simulink model "MainController"  (R2020a)
settings: Solver=VariableStepAuto  StartTime=0.0  StopTime=10.0  RelTol=1e-3
undefined symbols (not defined in the file): Angle, Ankle, Hip, Knee, Left, Right, Speed, Torque
settings Model: DataDictionary=MainControllerParameters.sldd  EnableAccessToBaseWorkspace=off  Creator=khoi  LastModifiedBy=khoi

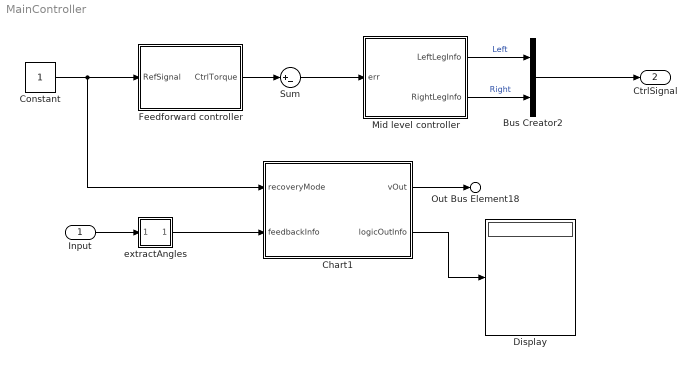
== system MainController ==
  Input : Inport  OutDataTypeStr=Bus: ExoskeletonSignal
  Bus Creator2 : BusCreator  Inputs=Left,Right  OutDataTypeStr=Bus: ExoskeletonSignal  NonVirtualBus=on
  Chart1 : Stateflow chart  TreatAsAtomicUnit=on
  Constant : Constant
  Display : Display
  Feedforward controller : Subsystem
  Mid level controller : Subsystem
  Sum : Sum  Inputs=|+-
  extractAngles : Subsystem
  Out Bus Element18 : Outport  PortName=Params  Element=vSupply
  CtrlSignal : Outport  Port=2
  wires:
  Sum/1 -> Mid level controller/1(err)
  Feedforward controller/1(CtrlTorque) -> Sum/1
  Constant/1 -> Chart1/1(recoveryMode), Feedforward controller/1(RefSignal)
  Chart1/1(vOut) -> Out Bus Element18/1
  Bus Creator2/1 -> CtrlSignal/1
  Mid level controller/2(RightLegInfo) -> Bus Creator2/2  "Right"
  Mid level controller/1(LeftLegInfo) -> Bus Creator2/1  "Left"
  Chart1/2(logicOutInfo) -> Display/1
  Input/1 -> extractAngles/1(In1)
  extractAngles/1(Out1) -> Chart1/2(feedbackInfo)

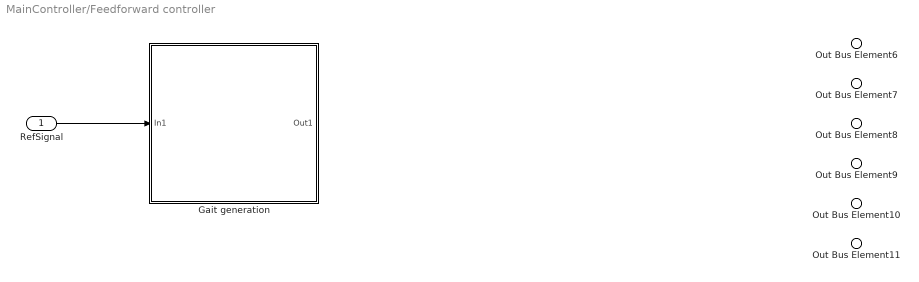
== system MainController/Feedforward controller ==
  RefSignal : Inport
  Gait generation : Subsystem
  Out Bus Element6 : Outport  PortName=CtrlTorque  Element=Left.Hip
  Out Bus Element8 : Outport  PortName=CtrlTorque  Element=Left.Knee
  Out Bus Element7 : Outport  PortName=CtrlTorque  Element=Left.Ankle
  Out Bus Element9 : Outport  PortName=CtrlTorque  Element=Right.Hip
  Out Bus Element10 : Outport  PortName=CtrlTorque  Element=Right.Knee
  Out Bus Element11 : Outport  PortName=CtrlTorque  Element=Right.Ankle
  wires:
  RefSignal/1 -> Gait generation/1(In1)

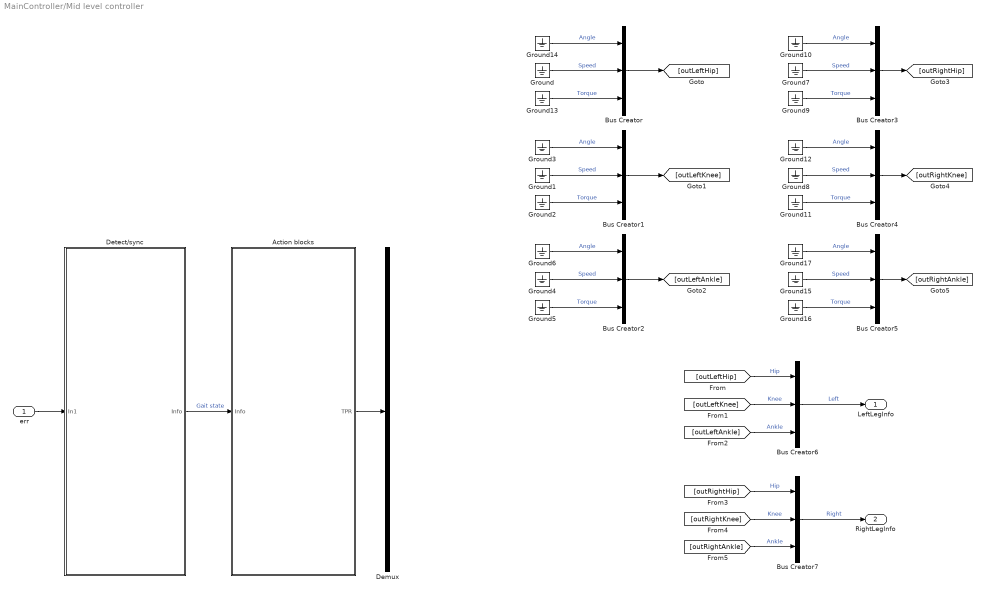
== system MainController/Mid level controller ==
  err : Inport
  Action blocks : Subsystem
  Bus Creator{,1..5} (6 alike) : BusCreator  Inputs=Angle,Speed,Torque  OutDataTypeStr=Bus: RespSignal  NonVirtualBus=on
  Bus Creator6 : BusCreator  Inputs=Hip,Knee,Ankle  OutDataTypeStr=Bus: LegSignal  NonVirtualBus=on
  Bus Creator7 : BusCreator  Inputs=Hip,Knee,Ankle  OutDataTypeStr=Bus: LegSignal  NonVirtualBus=on
  Demux : Demux  Outputs=6
  Detect/sync : Subsystem
  Ground{,1..17} (18 alike) : Ground
  LeftLegInfo : Outport
  RightLegInfo : Outport  Port=2
  wires:
  err/1 -> Detect/sync/1(In1)
  Detect/sync/1(Info) -> Action blocks/1(Info)  "Gait state"
  Action blocks/1(TPR) -> Demux/1
  Ground14/1 -> Bus Creator/1  "Angle"
  Ground/1 -> Bus Creator/2  "Speed"
  Ground13/1 -> Bus Creator/3  "Torque"
  Ground2/1 -> Bus Creator1/3  "Torque"
  Ground1/1 -> Bus Creator1/2  "Speed"
  Ground3/1 -> Bus Creator1/1  "Angle"
  Ground6/1 -> Bus Creator2/1  "Angle"
  Ground4/1 -> Bus Creator2/2  "Speed"
  Ground5/1 -> Bus Creator2/3  "Torque"
  Ground16/1 -> Bus Creator5/3  "Torque"
  Ground15/1 -> Bus Creator5/2  "Speed"
  Ground17/1 -> Bus Creator5/1  "Angle"
  Ground12/1 -> Bus Creator4/1  "Angle"
  Ground8/1 -> Bus Creator4/2  "Speed"
  Ground11/1 -> Bus Creator4/3  "Torque"
  Ground9/1 -> Bus Creator3/3  "Torque"
  Ground7/1 -> Bus Creator3/2  "Speed"
  Ground10/1 -> Bus Creator3/1  "Angle"
  Bus Creator/1 -> [outLeftHip]
  Bus Creator1/1 -> [outLeftKnee]
  Bus Creator2/1 -> [outLeftAnkle]
  Bus Creator3/1 -> [outRightHip]
  Bus Creator4/1 -> [outRightKnee]
  Bus Creator5/1 -> [outRightAnkle]
  [outLeftAnkle] -> Bus Creator6/3  "Ankle"
  [outRightHip] -> Bus Creator7/1  "Hip"
  [outLeftKnee] -> Bus Creator6/2  "Knee"
  [outLeftHip] -> Bus Creator6/1  "Hip"
  [outRightKnee] -> Bus Creator7/2  "Knee"
  [outRightAnkle] -> Bus Creator7/3  "Ankle"
  Bus Creator6/1 -> LeftLegInfo/1  "Left"
  Bus Creator7/1 -> RightLegInfo/1  "Right"

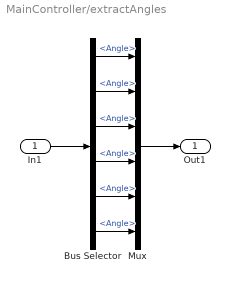
== system MainController/extractAngles ==
  In1 : Inport
  Bus Selector : BusSelector  OutputSignals=Left.Hip.Angle,Left.Knee.Angle,Left.Ankle.Angle,Right.Hip.Angle,Right.Knee.Angle,Right.Ankle.Angle
  Mux : Mux  Inputs=6
  Out1 : Outport
  wires:
  Bus Selector/4 -> Mux/4  "<Angle>"
  Bus Selector/6 -> Mux/6  "<Angle>"
  In1/1 -> Bus Selector/1
  Mux/1 -> Out1/1
  Bus Selector/1 -> Mux/1  "<Angle>"
  Bus Selector/5 -> Mux/5  "<Angle>"
  Bus Selector/3 -> Mux/3  "<Angle>"
  Bus Selector/2 -> Mux/2  "<Angle>"

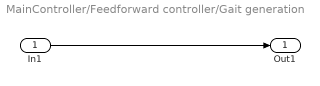
== system MainController/Feedforward controller/Gait generation ==
  In1 : Inport
  Out1 : Outport
  wires:
  In1/1 -> Out1/1

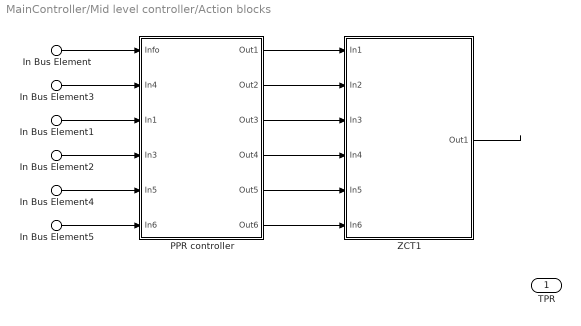
== system MainController/Mid level controller/Action blocks ==
  In Bus Element : Inport  PortName=Info  Element=Right.Hip
  In Bus Element1 : Inport  PortName=Info  Element=Right.Knee
  In Bus Element2 : Inport  PortName=Info  Element=Right.Ankle
  In Bus Element3 : Inport  PortName=Info  Element=Left.Hip
  In Bus Element4 : Inport  PortName=Info  Element=Left.Knee
  In Bus Element5 : Inport  PortName=Info  Element=Left.Ankle
  PPR controller : Subsystem
  ZCT1 : Subsystem
  TPR : Outport
  wires:
  ? -> TPR/1
  PPR controller/1(Out1) -> ZCT1/1(In1)
  ZCT1/1(Out1) -> ?
  In Bus Element/1 -> PPR controller/1(Info)
  In Bus Element3/1 -> PPR controller/2(In4)
  In Bus Element1/1 -> PPR controller/3(In1)
  In Bus Element2/1 -> PPR controller/4(In3)
  PPR controller/2(Out2) -> ZCT1/2(In2)
  PPR controller/3(Out3) -> ZCT1/3(In3)
  PPR controller/4(Out4) -> ZCT1/4(In4)
  In Bus Element4/1 -> PPR controller/5(In5)
  In Bus Element5/1 -> PPR controller/6(In6)
  PPR controller/5(Out5) -> ZCT1/5(In5)
  PPR controller/6(Out6) -> ZCT1/6(In6)

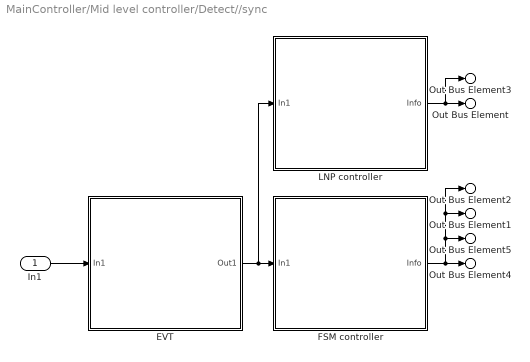
== system MainController/Mid level controller/Detect//sync ==
  In1 : Inport
  EVT : Subsystem
  FSM controller : Subsystem
  LNP controller : Subsystem
  Out Bus Element3 : Outport  PortName=Info  Element=Left.Hip
  Out Bus Element4 : Outport  PortName=Info  Element=Left.Knee
  Out Bus Element5 : Outport  PortName=Info  Element=Left.Ankle
  Out Bus Element : Outport  PortName=Info  Element=Right.Hip
  Out Bus Element1 : Outport  PortName=Info  Element=Right.Knee
  Out Bus Element2 : Outport  PortName=Info  Element=Right.Ankle
  wires:
  In1/1 -> EVT/1(In1)
  FSM controller/1(Info) -> Out Bus Element1/1, Out Bus Element2/1, Out Bus Element5/1, Out Bus Element4/1
  EVT/1(Out1) -> LNP controller/1(In1), FSM controller/1(In1)
  LNP controller/1(Info) -> Out Bus Element/1, Out Bus Element3/1

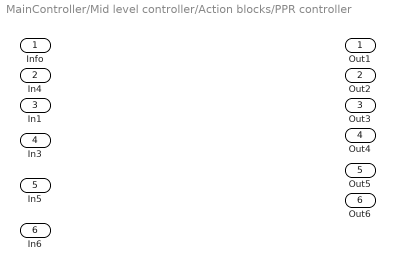
== system MainController/Mid level controller/Action blocks/PPR controller ==
  Info : Inport
  In4 : Inport  Port=2
  In1 : Inport  Port=3
  In3 : Inport  Port=4
  In5 : Inport  Port=5
  In6 : Inport  Port=6
  Out1 : Outport
  Out2 : Outport  Port=2
  Out3 : Outport  Port=3
  Out4 : Outport  Port=4
  Out5 : Outport  Port=5
  Out6 : Outport  Port=6

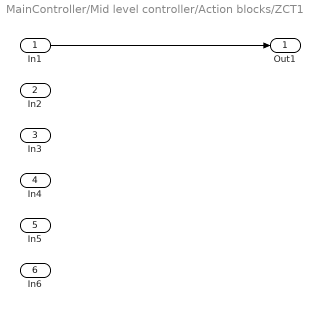
== system MainController/Mid level controller/Action blocks/ZCT1 ==
  In1 : Inport
  In2 : Inport  Port=2
  In3 : Inport  Port=3
  In4 : Inport  Port=4
  In5 : Inport  Port=5
  In6 : Inport  Port=6
  Out1 : Outport
  wires:
  In1/1 -> Out1/1

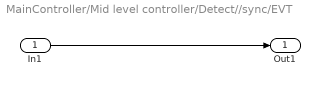
== system MainController/Mid level controller/Detect//sync/EVT ==
  In1 : Inport
  Out1 : Outport
  wires:
  In1/1 -> Out1/1

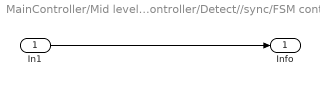
== system MainController/Mid level controller/Detect//sync/FSM controller ==
  In1 : Inport
  Info : Outport
  wires:
  In1/1 -> Info/1

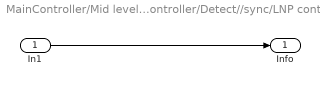
== system MainController/Mid level controller/Detect//sync/LNP controller ==
  In1 : Inport
  Info : Outport
  wires:
  In1/1 -> Info/1

== stateflow chart MainController/Chart1 ==
  state SITTING [group] [commented out]
  state GoToSitting [commented out]
  state ReadyForStandingUp [commented out]
  state InitParams
    entry:
    state voltageSupplyModifier
      (default) -> (junction 332) : % Control on patient's mobility
      (junction 332) -> (junction 333) [order 1] : [recoveryMode == 1]
      (junction 332) -> (junction 321) [order 2]
      (junction 333) -> (junction 334) : {vOut = 0.2*Vsup;}
      (junction 334) -> (junction 331)
      (junction 331) -> (junction 323)
      (junction 321) -> (junction 322) [order 1] : [recoveryMode == 2]
      (junction 321) -> (junction 325) [order 2]
      (junction 322) -> (junction 335) : {vOut = 0.4*Vsup;}
      (junction 335) -> (junction 323)
      (junction 323) -> (junction 319)
      (junction 325) -> (junction 326) [order 1] : [recoveryMode == 3]
      (junction 325) -> (junction 320) [order 2]
      (junction 326) -> (junction 328) : {vOut = 0.6*Vsup;}
      (junction 328) -> (junction 319)
      (junction 319) -> (junction 351)
      (junction 320) -> (junction 329) [order 1] : [recoveryMode == 4]
      (junction 320) -> (junction 350) [order 2]
      (junction 329) -> (junction 330) : {vOut = 0.8*Vsup;}
      (junction 330) -> (junction 351)
      (junction 351) -> (junction 349)
      (junction 350) -> (junction 352) [order 1] : [recoveryMode == 5]
      (junction 350) -> (junction 353) [order 2] : {vOut = 0;}
      (junction 352) -> (junction 346) : {vOut = 1.0*Vsup;}
      (junction 346) -> (junction 349)
      (junction 349) -> (junction 354)
      (junction 354) -> (junction 353)
      (junction 353) -> (junction 345)
    state dataOut
      entry:
      %logicOutInfo = feedbackInfo > [1 2 3 4 5 6]';
      logicOutInfo = feedbackInfo;
    (default) -> voltageSupplyModifier
    voltageSupplyModifier -> dataOut
  state STANDING_READY [group] [commented out]
  state SittingDown [commented out]
  state STANDING [group] [commented out]
  state GoToStanding [commented out]
  state StandingUp [commented out]
  state RightBackwardToStanding [commented out]
  state LeftForwardToStanding [commented out]
  state LeftStep [commented out]
  state RightStep [commented out]
  state LEFT_FORWARD [group] [commented out]
  state DoubleStand_in_LeftForward [commented out]
  state DoubleStand_RightSwing [commented out]
  state RIGHT_FORWARD [group] [commented out]
  state RightStand_LeftSwing [commented out]
  state DoubleStand_in_RightForward [commented out]
  SITTING -> ReadyForStandingUp [commented out]
  GoToSitting -> SITTING [commented out]
  (default) -> GoToSitting [commented out]
  ReadyForStandingUp -> STANDING_READY [commented out]
  (default) -> InitParams
  SittingDown -> SITTING [commented out]
  STANDING -> SittingDown [commented out]
  (default) -> GoToStanding [commented out]
  STANDING_READY -> StandingUp [commented out]
  GoToStanding -> STANDING [commented out]
  StandingUp -> STANDING [commented out]
  RightBackwardToStanding -> STANDING [commented out]
  LeftForwardToStanding -> STANDING [commented out]
  STANDING -> LeftStep [commented out]
  STANDING -> RightStep [commented out]
  RIGHT_FORWARD -> RightBackwardToStanding [commented out]
  RightStep -> RIGHT_FORWARD [commented out]
  LEFT_FORWARD -> LeftForwardToStanding [commented out]
  LeftStep -> LEFT_FORWARD [commented out]
  DoubleStand_in_LeftForward -> DoubleStand_RightSwing [commented out]
  LEFT_FORWARD -> DoubleStand_in_LeftForward [commented out]
  DoubleStand_RightSwing -> RIGHT_FORWARD [commented out]
  RightStand_LeftSwing -> LEFT_FORWARD [commented out]
  DoubleStand_in_RightForward -> RightStand_LeftSwing [commented out]
  RIGHT_FORWARD -> DoubleStand_in_RightForward [commented out]
  data: recoveryMode input; Vsup constant double =24; vOut output; initBoot local; feedbackInfo input; logicOutInfo output
